simulink model "hmedidobackup"  (R2021a)
settings: Solver=VariableStepAuto  StartTime=0.0  StopTime=10.0  RelTol=1e-3
values from neighbouring files (symbols this model uses):
  a1 = 0.15    [a.m]
  a2 = 0.2    [a.m]
  b1 = 0.3    [a.m]
  b2 = 0.5    [a.m]
settings Model: Creator=valen  LastModifiedBy=valen

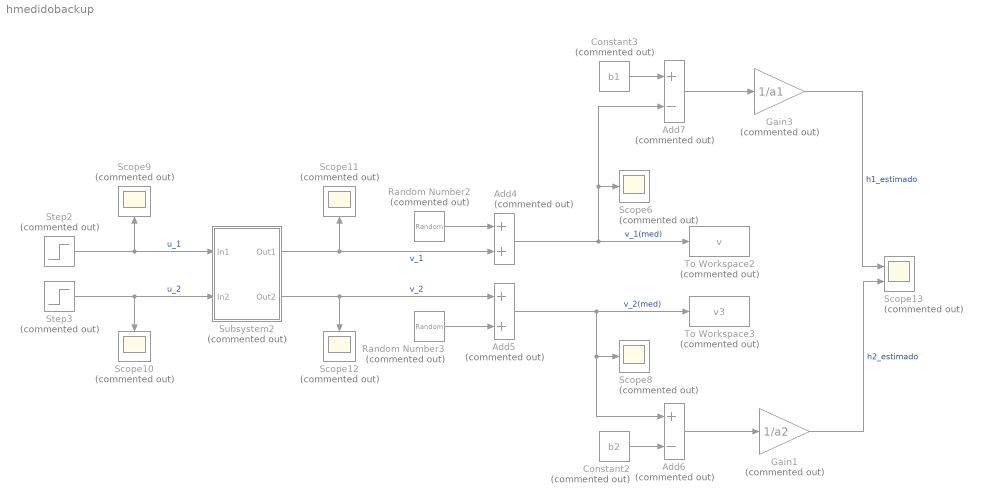
== system hmedidobackup ==
  Add4 : Sum  Commented=on
  Add5 : Sum  Commented=on
  Add6 : Sum  Commented=on  Inputs=+-
  Add7 : Sum  Commented=on  Inputs=+-
  Constant2 : Constant  Commented=on  Value=b2
  Constant3 : Constant  Commented=on  Value=b1
  Gain1 : Gain  Commented=on  Gain=1/a2
  Gain3 : Gain  Commented=on  Gain=1/a1
  Random Number2 : RandomNumber  Commented=on  Variance=1e-6  SampleTime=0.1
  Random Number3 : RandomNumber  Commented=on  Variance=1e-6  SampleTime=0.1
  Scope{6,8..12} (6 alike) : Scope  Commented=on
  Scope13 : Scope  Commented=on  NumInputPorts=2
  Step2 : Step  Commented=on  After=0  SampleTime=0
  Step3 : Step  Commented=on  After=0  SampleTime=0
  Subsystem2 : Subsystem  Commented=on  mask{a1=0.15, a2=0.2, b1=0.3, b2=0.5, c1=0.3, c2=-0.4, d1=6, d2=20}
  To Workspace2 : ToWorkspace  Commented=on  VariableName=v  SaveFormat=Timeseries  SampleTime=-1
  To Workspace3 : ToWorkspace  Commented=on  VariableName=v3  SaveFormat=Timeseries  SampleTime=-1
  wires:
  Step2/1 -> Scope9/1, Subsystem2/1(In1)  "u_1"
  Subsystem2/1(Out1) -> Add4/2, Scope11/1  "v_1"
  Add5/1 -> To Workspace3/1, Scope8/1, Add6/1  "v_2(med)"
  Step3/1 -> Scope10/1, Subsystem2/2(In2)  "u_2"
  Random Number3/1 -> Add5/2
  Subsystem2/2(Out2) -> Add5/1, Scope12/1  "v_2"
  Add6/1 -> Gain1/1
  Gain3/1 -> Scope13/1  "h1_estimado"
  Add7/1 -> Gain3/1
  Constant2/1 -> Add6/2
  Gain1/1 -> Scope13/2  "h2_estimado"
  Random Number2/1 -> Add4/1
  Add4/1 -> Add7/2, Scope6/1, To Workspace2/1  "v_1(med)"
  Constant3/1 -> Add7/1

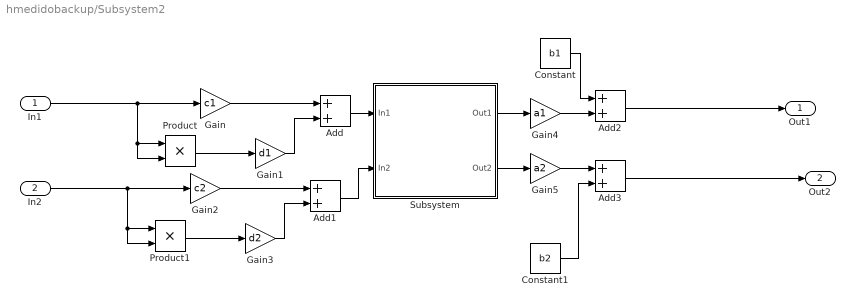
== system hmedidobackup/Subsystem2 ==
  In1 : Inport
  In2 : Inport  Port=2
  Add{,1..3} (4 alike) : Sum
  Constant : Constant  Value=b1
  Constant1 : Constant  Value=b2
  Gain : Gain  Gain=c1
  Gain1 : Gain  Gain=d1
  Gain2 : Gain  Gain=c2
  Gain3 : Gain  Gain=d2
  Gain4 : Gain  Gain=a1
  Gain5 : Gain  Gain=a2
  Product : Product
  Product1 : Product
  Subsystem : Subsystem  mask{A=100, K=15, h10=20, h20=10}
      mask prompts: A "Area"; h10 "Altura Inicial 1"; h20 "Altura Inicial 2"
  Out1 : Outport
  Out2 : Outport  Port=2
  wires:
  Add3/1 -> Out2/1
  Subsystem/1(Out1) -> Gain4/1
  In2/1 -> Product1/1, Product1/2, Gain2/1
  Constant/1 -> Add2/1
  Gain5/1 -> Add3/1
  Gain3/1 -> Add1/2
  Constant1/1 -> Add3/2
  In1/1 -> Product/2, Product/1, Gain/1
  Gain/1 -> Add/1
  Subsystem/2(Out2) -> Gain5/1
  Product1/1 -> Gain3/1
  Gain2/1 -> Add1/1
  Add1/1 -> Subsystem/2(In2)
  Add2/1 -> Out1/1
  Product/1 -> Gain1/1
  Gain4/1 -> Add2/2
  Gain1/1 -> Add/2
  Add/1 -> Subsystem/1(In1)

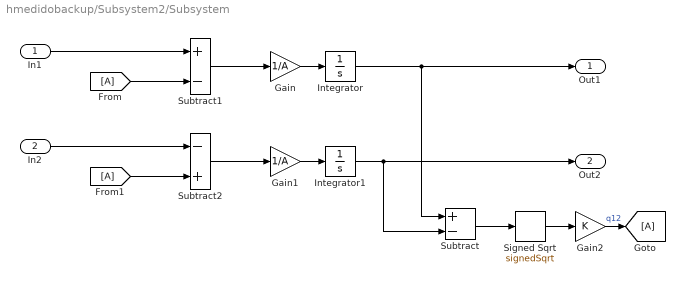
== system hmedidobackup/Subsystem2/Subsystem ==
  In1 : Inport
  In2 : Inport  Port=2
  Gain : Gain  Gain=1/A
  Gain1 : Gain  Gain=1/A
  Gain2 : Gain  Gain=K
  Integrator : Integrator  InitialCondition=h10
  Integrator1 : Integrator  InitialCondition=h20
  Signed Sqrt : Sqrt  Operator=signedSqrt  SaturateOnIntegerOverflow=on
  Subtract : Sum  Inputs=+-
  Subtract1 : Sum  Inputs=+-
  Subtract2 : Sum  Inputs=-+
  Out1 : Outport
  Out2 : Outport  Port=2
  wires:
  In2/1 -> Subtract2/1
  [A] -> Subtract2/2
  Gain/1 -> Integrator/1
  [A] -> Subtract1/2
  Subtract/1 -> Signed Sqrt/1
  Integrator/1 -> Out1/1, Subtract/1
  Signed Sqrt/1 -> Gain2/1
  Integrator1/1 -> Out2/1, Subtract/2
  Subtract2/1 -> Gain1/1
  Gain2/1 -> [A]  "q12"
  In1/1 -> Subtract1/1
  Gain1/1 -> Integrator1/1
  Subtract1/1 -> Gain/1
